simulink model "solpos"  (R2026a)
settings: Solver=FixedStepAuto  StopTime=365*24*3600  FixedStep=600
settings Model: Creator=cdt  LastModifiedBy=cdt

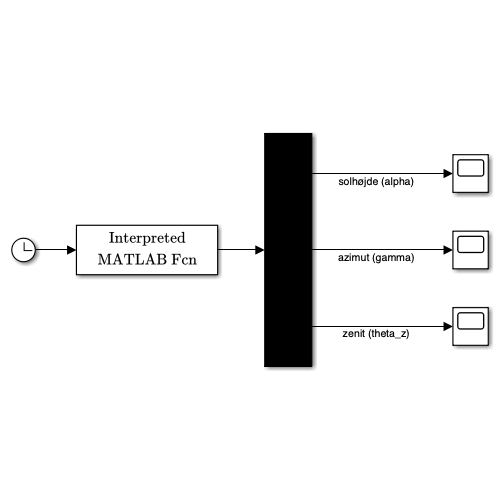
[thumbnail: Simulink's stored preview of the top-level diagram]
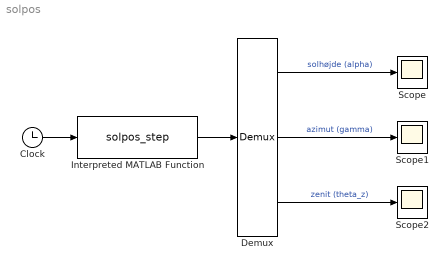
== system solpos ==
  Clock : Clock
  Demux : Demux  Outputs=3
  Interpreted MATLAB Function : MATLABFcn  MATLABFcn=solpos_step  OutputDimensions=3
  Scope : Scope
      settings: ActiveDisplayYMinimum=-70.4853872876399  ActiveDisplayYMaximum=70.485585804842628
  Scope1 : Scope
      settings: ActiveDisplayYMinimum=-44.998583681912983  ActiveDisplayYMaximum=404.9895260680355
  Scope2 : Scope
      settings: ActiveDisplayYMinimum=19.514414195157368  ActiveDisplayYMaximum=160.4853872876399  DataLoggingVariableName=ScopeData2
  wires:
  Clock/1 -> Interpreted MATLAB Function/1
  Demux/1 -> Scope/1  "solhøjde (alpha)"
  Demux/2 -> Scope1/1  "azimut (gamma)"
  Demux/3 -> Scope2/1  "zenit (theta_z)"
  Interpreted MATLAB Function/1 -> Demux/1
